simulink model "Dynamics"  (R2018a)
settings: Solver=FixedStepDiscrete  StartTime=0.0  StopTime=10.0  FixedStep=Ts  RelTol=1e-3
undefined symbols (not defined in the file): Ts
libraries: aerolibutil x5, vrlib x4
settings Model: Creator=henry  LastModifiedBy=henry

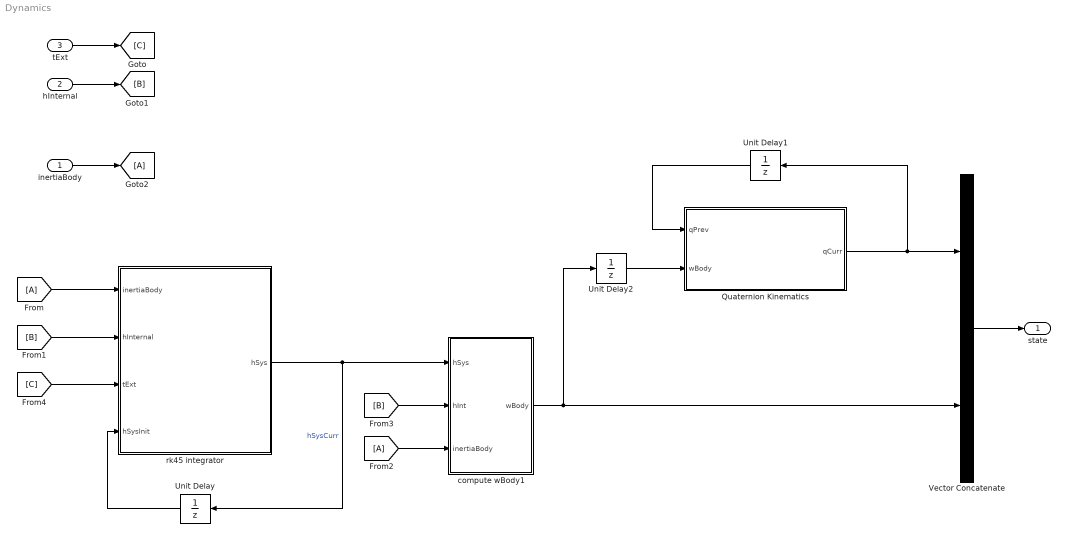
== system Dynamics ==
  inertiaBody : Inport  OutDataTypeStr=Bus: DynamicsInput
  hInternal : Inport  Port=2  OutDataTypeStr=Bus: massProperties
  tExt : Inport  Port=3
  Quaternion Kinematics : Subsystem
  Unit Delay : UnitDelay  InitialCondition=[1 1 1]  SampleTime=-1
  Unit Delay1 : UnitDelay  InitialCondition=[1 2 3 4]  SampleTime=-1
  Unit Delay2 : UnitDelay  InitialCondition=[1 1 1]  SampleTime=-1
  Vector Concatenate : Concatenate
  compute wBody1 : Subsystem
  rk45 integrator : Subsystem
  "state " : Outport
  wires:
  [A] -> compute wBody1/3(inertiaBody)
  [B] -> compute wBody1/2(hInt)
  rk45 integrator/1(hSys) -> Unit Delay/1, compute wBody1/1(hSys)  "hSysCurr"
  Quaternion Kinematics/1(qCurr) -> Unit Delay1/1, Vector Concatenate/1
  compute wBody1/1(wBody) -> Unit Delay2/1, Vector Concatenate/2
  Unit Delay/1 -> rk45 integrator/4(hSysInit)
  Unit Delay1/1 -> Quaternion Kinematics/1(qPrev)
  Unit Delay2/1 -> Quaternion Kinematics/2(wBody)
  Vector Concatenate/1 -> "state "/1
  [A] -> rk45 integrator/1(inertiaBody)
  [B] -> rk45 integrator/2(hInternal)
  [C] -> rk45 integrator/3(tExt)
  inertiaBody/1 -> [A]
  tExt/1 -> [C]
  hInternal/1 -> [B]

== system Dynamics/Quaternion Kinematics ==
  qPrev : Inport
  wBody : Inport  Port=2
  Terminator : Terminator
  "crossMatrix " : Subsystem  mask(Cross Matrix){}
      mask help: This block takes in a 3x1 vector and outputs it's corresponding 3x3 cross product matrix
  qCurr : Outport
  wires:
  qPrev/1 -> qCurr/1
  wBody/1 -> Terminator/1

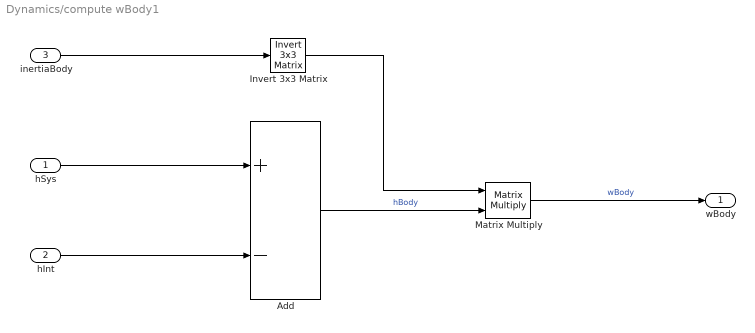
== system Dynamics/compute wBody1 ==
  hSys : Inport
  hInt : Inport  Port=2
  inertiaBody : Inport  Port=3  OutDataTypeStr=double
  Add : Sum  Inputs=+-
  Invert 3x3 Matrix : aerolibutil/Invert  3x3 Matrix
  Matrix Multiply : Product  Multiplication=Matrix(*)
  wBody : Outport
  wires:
  Add/1 -> Matrix Multiply/2  "hBody"
  hInt/1 -> Add/2
  Invert 3x3 Matrix/1 -> Matrix Multiply/1
  Matrix Multiply/1 -> wBody/1  "wBody"
  hSys/1 -> Add/1
  inertiaBody/1 -> Invert 3x3 Matrix/1

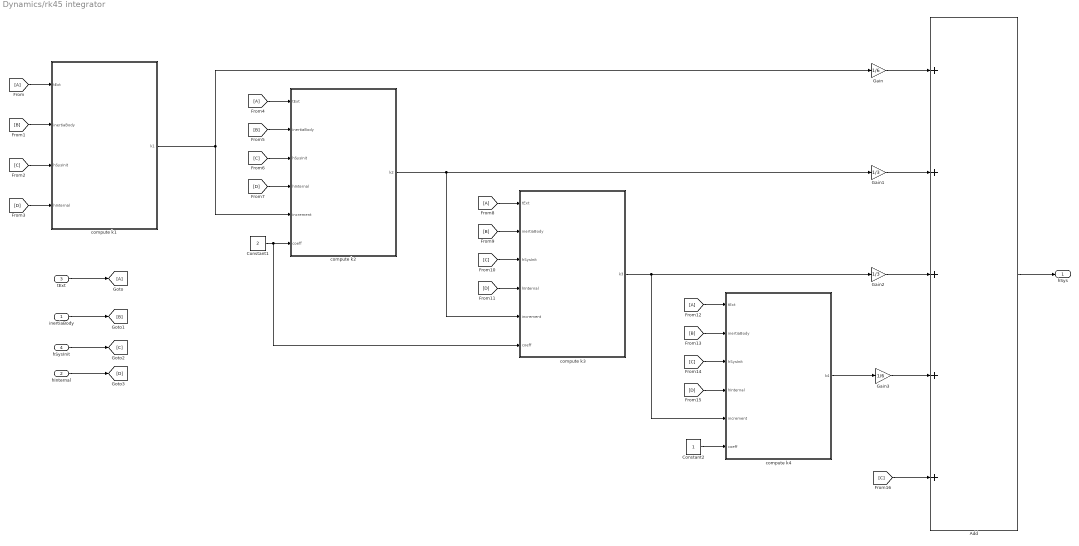
== system Dynamics/rk45 integrator ==
  inertiaBody : Inport
  hInternal : Inport  Port=2
  tExt : Inport  Port=3
  hSysInit : Inport  Port=4
  Add : Sum  Inputs=+++++
  Constant1 : Constant  Value=2
  Constant2 : Constant
  Gain : Gain  Gain=1/6
  Gain1 : Gain  Gain=1/3
  Gain2 : Gain  Gain=1/3
  Gain3 : Gain  Gain=1/6
  compute k1 : Subsystem
  compute k2 : Subsystem
  compute k3 : Subsystem
  compute k4 : Subsystem
  hSys : Outport
  wires:
  [A] -> compute k1/1(tExt)
  tExt/1 -> [A]
  inertiaBody/1 -> [B]
  hSysInit/1 -> [C]
  hInternal/1 -> [D]
  [B] -> compute k1/2(inertiaBody)
  [C] -> compute k1/3(hSysInit)
  [D] -> compute k1/4(hInternal)
  [B] -> compute k2/2(inertiaBody)
  [D] -> compute k2/4(hInternal)
  [A] -> compute k2/1(tExt)
  [C] -> compute k2/3(hSysInit)
  [B] -> compute k3/2(inertiaBody)
  [D] -> compute k3/4(hInternal)
  [A] -> compute k3/1(tExt)
  [C] -> compute k3/3(hSysInit)
  [B] -> compute k4/2(inertiaBody)
  [D] -> compute k4/4(hInternal)
  [A] -> compute k4/1(tExt)
  [C] -> compute k4/3(hSysInit)
  compute k1/1(k1) -> Gain/1, compute k2/5(increment)
  compute k2/1(k2) -> compute k3/5(increment), Gain1/1
  compute k3/1(k3) -> compute k4/5(increment), Gain2/1
  Constant2/1 -> compute k4/6(coeff)
  Constant1/1 -> compute k3/6(coeff), compute k2/6(coeff)
  compute k4/1(k4) -> Gain3/1
  Gain/1 -> Add/1
  Gain1/1 -> Add/2
  Gain2/1 -> Add/3
  Gain3/1 -> Add/4
  [C] -> Add/5
  Add/1 -> hSys/1

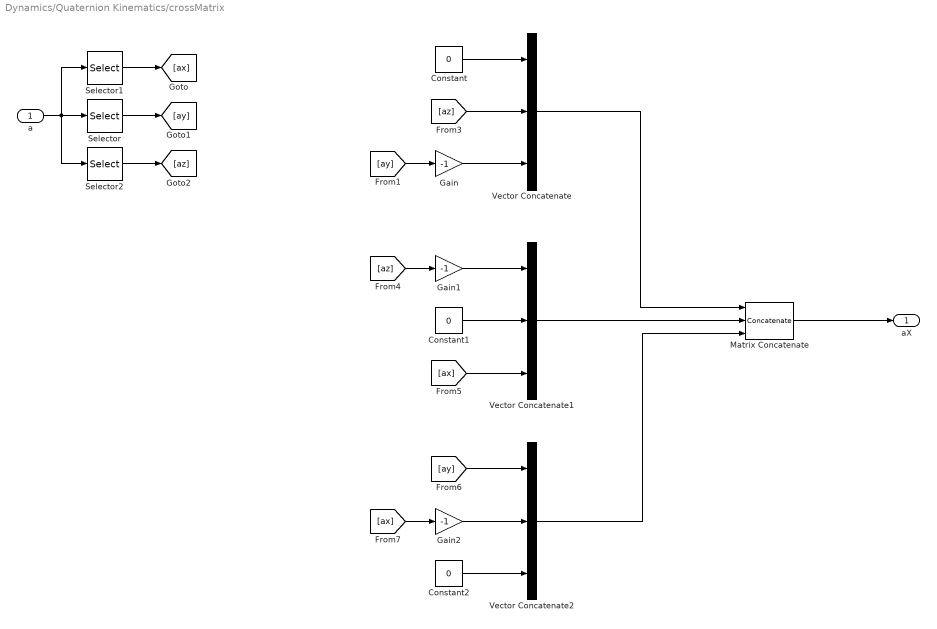
== system Dynamics/Quaternion Kinematics/crossMatrix  ==
  a : Inport
  Constant : Constant  Value=0
  Constant1 : Constant  Value=0
  Constant2 : Constant  Value=0
  Gain : Gain  Gain=-1
  Gain1 : Gain  Gain=-1
  Gain2 : Gain  Gain=-1
  Matrix Concatenate : Concatenate  NumInputs=3  Mode=Multidimensional array  ConcatenateDimension=2
  Selector : Selector  InputPortWidth=3  IndexOptions=Index vector (dialog)  Indices=2  OutputSizes=1
  Selector1 : Selector  InputPortWidth=3  IndexOptions=Index vector (dialog)  Indices=1  OutputSizes=1
  Selector2 : Selector  InputPortWidth=3  IndexOptions=Index vector (dialog)  Indices=3  OutputSizes=1
  Vector Concatenate : Concatenate  NumInputs=3
  Vector Concatenate1 : Concatenate  NumInputs=3
  Vector Concatenate2 : Concatenate  NumInputs=3
  aX : Outport
  wires:
  [ay] -> Gain/1
  [az] -> Gain1/1
  Gain2/1 -> Vector Concatenate2/2
  Constant1/1 -> Vector Concatenate1/2
  [ax] -> Vector Concatenate1/3
  [ay] -> Vector Concatenate2/1
  Vector Concatenate1/1 -> Matrix Concatenate/2
  Matrix Concatenate/1 -> aX/1
  Constant2/1 -> Vector Concatenate2/3
  [ax] -> Gain2/1
  Vector Concatenate2/1 -> Matrix Concatenate/3
  Gain/1 -> Vector Concatenate/3
  Vector Concatenate/1 -> Matrix Concatenate/1
  Selector1/1 -> [ax]
  Selector2/1 -> [az]
  [az] -> Vector Concatenate/2
  Gain1/1 -> Vector Concatenate1/1
  Constant/1 -> Vector Concatenate/1
  a/1 -> Selector/1, Selector1/1, Selector2/1
  Selector/1 -> [ay]

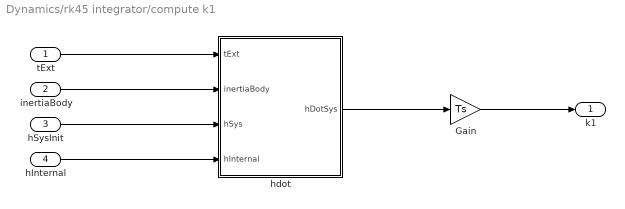
== system Dynamics/rk45 integrator/compute k1 ==
  tExt : Inport
  inertiaBody : Inport  Port=2
  hSysInit : Inport  Port=3
  hInternal : Inport  Port=4
  Gain : Gain  Gain=Ts
  hdot : Subsystem
  k1 : Outport
  wires:
  hInternal/1 -> hdot/4(hInternal)
  inertiaBody/1 -> hdot/2(inertiaBody)
  tExt/1 -> hdot/1(tExt)
  hdot/1(hDotSys) -> Gain/1
  Gain/1 -> k1/1
  hSysInit/1 -> hdot/3(hSys)

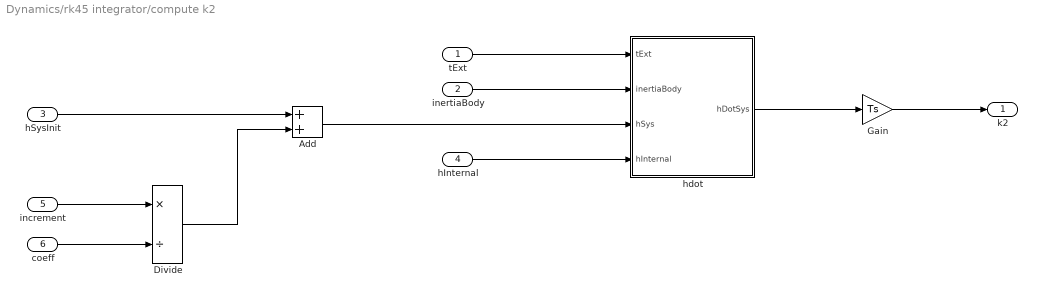
== system Dynamics/rk45 integrator/compute k2 ==
  tExt : Inport
  inertiaBody : Inport  Port=2
  hSysInit : Inport  Port=3
  hInternal : Inport  Port=4
  increment : Inport  Port=5
  coeff : Inport  Port=6
  Add : Sum
  Divide : Product  Inputs=*/
  Gain : Gain  Gain=Ts
  hdot : Subsystem
  k2 : Outport
  wires:
  hInternal/1 -> hdot/4(hInternal)
  inertiaBody/1 -> hdot/2(inertiaBody)
  tExt/1 -> hdot/1(tExt)
  hSysInit/1 -> Add/1
  increment/1 -> Divide/1
  coeff/1 -> Divide/2
  Divide/1 -> Add/2
  Add/1 -> hdot/3(hSys)
  hdot/1(hDotSys) -> Gain/1
  Gain/1 -> k2/1

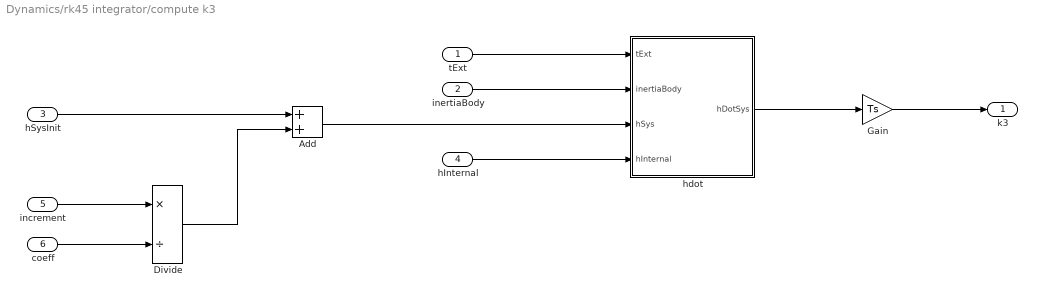
== system Dynamics/rk45 integrator/compute k3 ==
  tExt : Inport
  inertiaBody : Inport  Port=2
  hSysInit : Inport  Port=3
  hInternal : Inport  Port=4
  increment : Inport  Port=5
  coeff : Inport  Port=6
  Add : Sum
  Divide : Product  Inputs=*/
  Gain : Gain  Gain=Ts
  hdot : Subsystem
  k3 : Outport
  wires:
  hInternal/1 -> hdot/4(hInternal)
  inertiaBody/1 -> hdot/2(inertiaBody)
  tExt/1 -> hdot/1(tExt)
  hSysInit/1 -> Add/1
  increment/1 -> Divide/1
  coeff/1 -> Divide/2
  Divide/1 -> Add/2
  Add/1 -> hdot/3(hSys)
  hdot/1(hDotSys) -> Gain/1
  Gain/1 -> k3/1

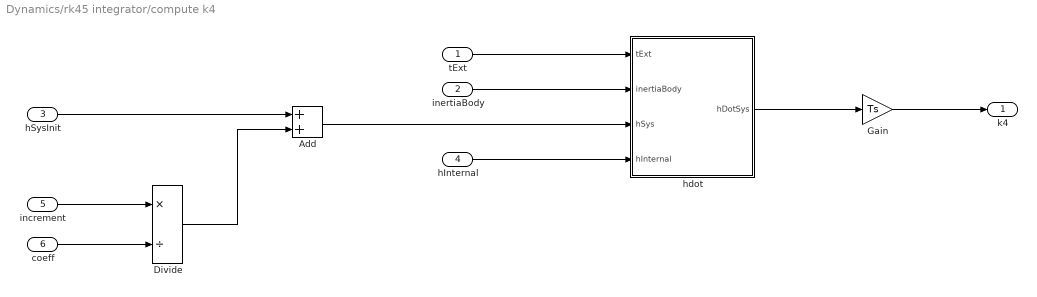
== system Dynamics/rk45 integrator/compute k4 ==
  tExt : Inport
  inertiaBody : Inport  Port=2
  hSysInit : Inport  Port=3
  hInternal : Inport  Port=4
  increment : Inport  Port=5
  coeff : Inport  Port=6
  Add : Sum
  Divide : Product  Inputs=*/
  Gain : Gain  Gain=Ts
  hdot : Subsystem
  k4 : Outport
  wires:
  hInternal/1 -> hdot/4(hInternal)
  inertiaBody/1 -> hdot/2(inertiaBody)
  tExt/1 -> hdot/1(tExt)
  hSysInit/1 -> Add/1
  increment/1 -> Divide/1
  coeff/1 -> Divide/2
  Divide/1 -> Add/2
  Add/1 -> hdot/3(hSys)
  hdot/1(hDotSys) -> Gain/1
  Gain/1 -> k4/1

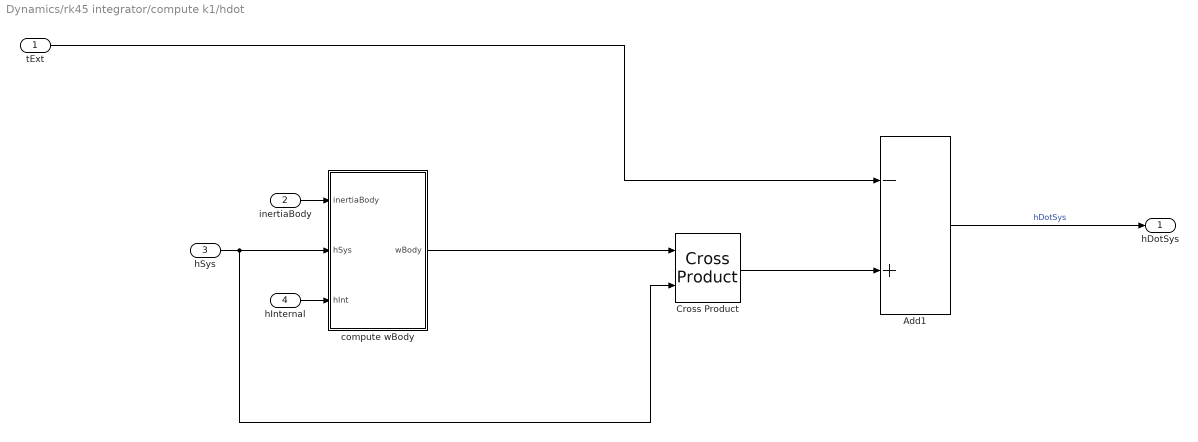
== system Dynamics/rk45 integrator/compute k1/hdot ==
  tExt : Inport
  inertiaBody : Inport  Port=2
  hSys : Inport  Port=3
  hInternal : Inport  Port=4
  Add1 : Sum  Inputs=-+
  Cross Product : vrlib/Utilities/Cross Product
      settings: SourceProductBaseCode=VR
  compute wBody : Subsystem
  hDotSys : Outport
  wires:
  Add1/1 -> hDotSys/1  "hDotSys"
  tExt/1 -> Add1/1
  Cross Product/1 -> Add1/2
  inertiaBody/1 -> compute wBody/1(inertiaBody)
  hInternal/1 -> compute wBody/3(hInt)
  compute wBody/1(wBody) -> Cross Product/1
  hSys/1 -> Cross Product/2, compute wBody/2(hSys)

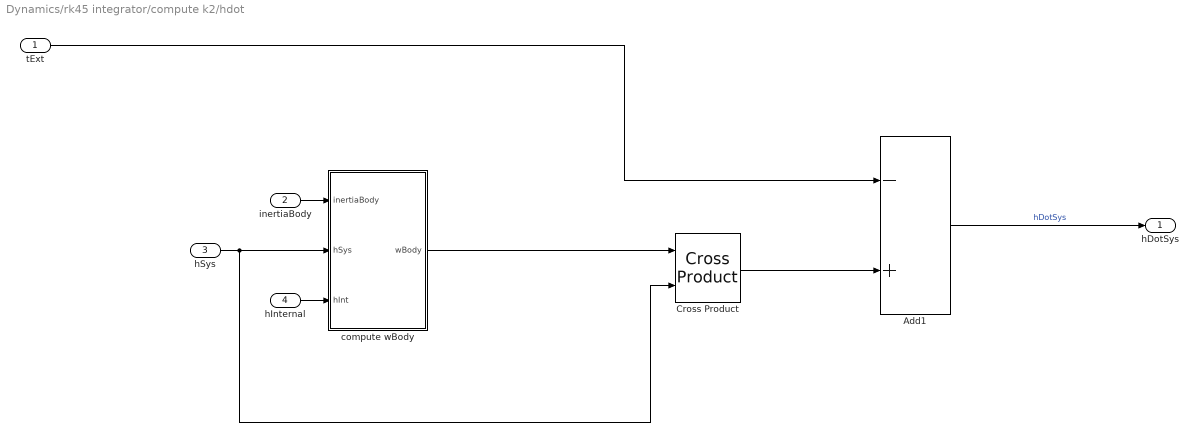
== system Dynamics/rk45 integrator/compute k2/hdot ==
  tExt : Inport
  inertiaBody : Inport  Port=2
  hSys : Inport  Port=3
  hInternal : Inport  Port=4
  Add1 : Sum  Inputs=-+
  Cross Product : vrlib/Utilities/Cross Product
      settings: SourceProductBaseCode=VR
  compute wBody : Subsystem
  hDotSys : Outport
  wires:
  Add1/1 -> hDotSys/1  "hDotSys"
  tExt/1 -> Add1/1
  Cross Product/1 -> Add1/2
  inertiaBody/1 -> compute wBody/1(inertiaBody)
  hInternal/1 -> compute wBody/3(hInt)
  compute wBody/1(wBody) -> Cross Product/1
  hSys/1 -> Cross Product/2, compute wBody/2(hSys)

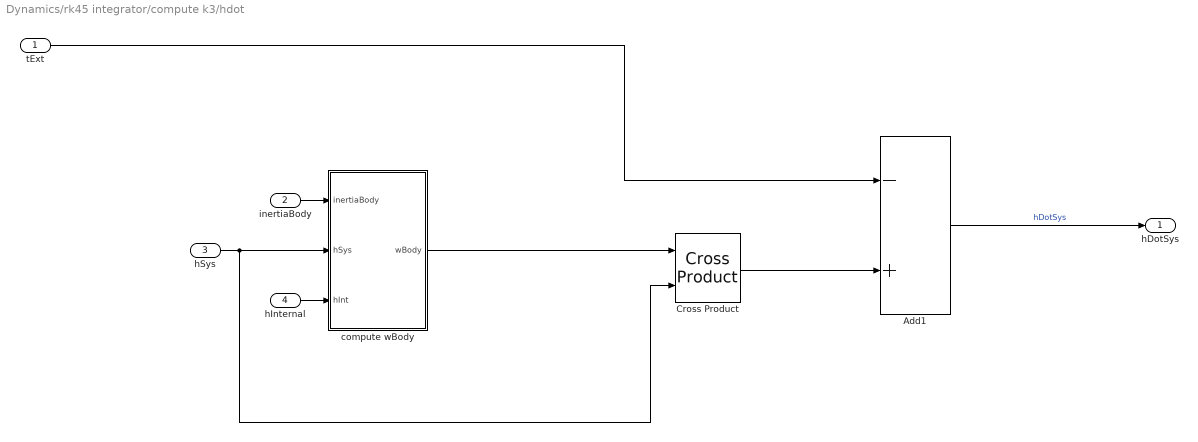
== system Dynamics/rk45 integrator/compute k3/hdot ==
  tExt : Inport
  inertiaBody : Inport  Port=2
  hSys : Inport  Port=3
  hInternal : Inport  Port=4
  Add1 : Sum  Inputs=-+
  Cross Product : vrlib/Utilities/Cross Product
      settings: SourceProductBaseCode=VR
  compute wBody : Subsystem
  hDotSys : Outport
  wires:
  Add1/1 -> hDotSys/1  "hDotSys"
  tExt/1 -> Add1/1
  Cross Product/1 -> Add1/2
  inertiaBody/1 -> compute wBody/1(inertiaBody)
  hInternal/1 -> compute wBody/3(hInt)
  compute wBody/1(wBody) -> Cross Product/1
  hSys/1 -> Cross Product/2, compute wBody/2(hSys)

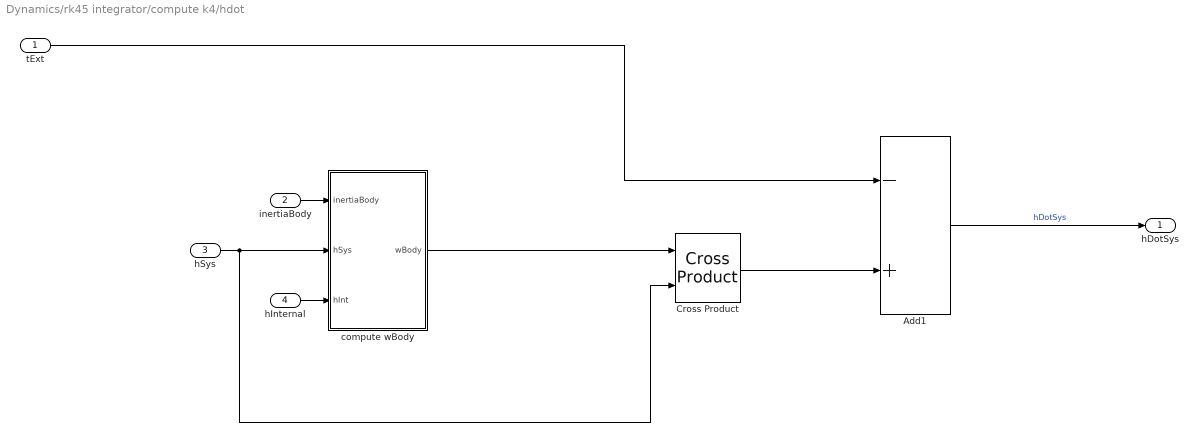
== system Dynamics/rk45 integrator/compute k4/hdot ==
  tExt : Inport
  inertiaBody : Inport  Port=2
  hSys : Inport  Port=3
  hInternal : Inport  Port=4
  Add1 : Sum  Inputs=-+
  Cross Product : vrlib/Utilities/Cross Product
      settings: SourceProductBaseCode=VR
  compute wBody : Subsystem
  hDotSys : Outport
  wires:
  Add1/1 -> hDotSys/1  "hDotSys"
  tExt/1 -> Add1/1
  Cross Product/1 -> Add1/2
  inertiaBody/1 -> compute wBody/1(inertiaBody)
  hInternal/1 -> compute wBody/3(hInt)
  compute wBody/1(wBody) -> Cross Product/1
  hSys/1 -> Cross Product/2, compute wBody/2(hSys)

== system Dynamics/rk45 integrator/compute k1/hdot/compute wBody ==
  inertiaBody : Inport
  hSys : Inport  Port=2
  hInt : Inport  Port=3
  Add : Sum  Inputs=+-
  Invert 3x3 Matrix : aerolibutil/Invert  3x3 Matrix
  Matrix Multiply : Product  Multiplication=Matrix(*)
  wBody : Outport
  wires:
  inertiaBody/1 -> Invert 3x3 Matrix/1
  hSys/1 -> Add/1
  Matrix Multiply/1 -> wBody/1  "wBody"
  Invert 3x3 Matrix/1 -> Matrix Multiply/1
  hInt/1 -> Add/2
  Add/1 -> Matrix Multiply/2  "hBody"

== system Dynamics/rk45 integrator/compute k2/hdot/compute wBody ==
  inertiaBody : Inport
  hSys : Inport  Port=2
  hInt : Inport  Port=3
  Add : Sum  Inputs=+-
  Invert 3x3 Matrix : aerolibutil/Invert  3x3 Matrix
  Matrix Multiply : Product  Multiplication=Matrix(*)
  wBody : Outport
  wires:
  inertiaBody/1 -> Invert 3x3 Matrix/1
  hSys/1 -> Add/1
  Matrix Multiply/1 -> wBody/1  "wBody"
  Invert 3x3 Matrix/1 -> Matrix Multiply/1
  hInt/1 -> Add/2
  Add/1 -> Matrix Multiply/2  "hBody"

== system Dynamics/rk45 integrator/compute k3/hdot/compute wBody ==
  inertiaBody : Inport
  hSys : Inport  Port=2
  hInt : Inport  Port=3
  Add : Sum  Inputs=+-
  Invert 3x3 Matrix : aerolibutil/Invert  3x3 Matrix
  Matrix Multiply : Product  Multiplication=Matrix(*)
  wBody : Outport
  wires:
  inertiaBody/1 -> Invert 3x3 Matrix/1
  hSys/1 -> Add/1
  Matrix Multiply/1 -> wBody/1  "wBody"
  Invert 3x3 Matrix/1 -> Matrix Multiply/1
  hInt/1 -> Add/2
  Add/1 -> Matrix Multiply/2  "hBody"

== system Dynamics/rk45 integrator/compute k4/hdot/compute wBody ==
  inertiaBody : Inport
  hSys : Inport  Port=2
  hInt : Inport  Port=3
  Add : Sum  Inputs=+-
  Invert 3x3 Matrix : aerolibutil/Invert  3x3 Matrix
  Matrix Multiply : Product  Multiplication=Matrix(*)
  wBody : Outport
  wires:
  inertiaBody/1 -> Invert 3x3 Matrix/1
  hSys/1 -> Add/1
  Matrix Multiply/1 -> wBody/1  "wBody"
  Invert 3x3 Matrix/1 -> Matrix Multiply/1
  hInt/1 -> Add/2
  Add/1 -> Matrix Multiply/2  "hBody"
